simulink model "simulinkModelForOpenLoop"  (R2020b)
settings: Solver=VariableStepAuto  StartTime=0.0  StopTime=10.0  RelTol=1e-3
settings Model: Creator=saumya  LastModifiedBy=saumya

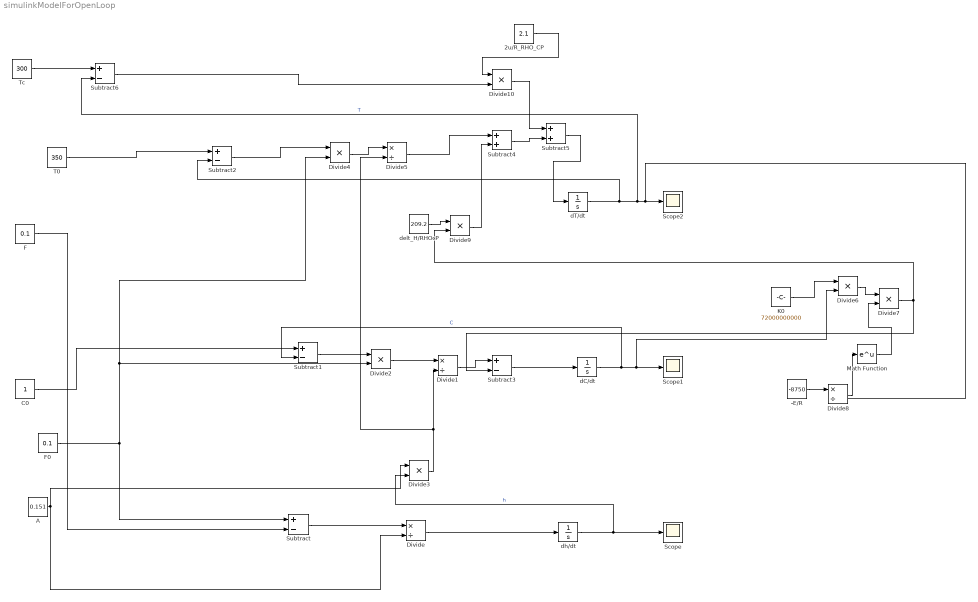
== system simulinkModelForOpenLoop ==
  -E/R : Constant  Value=-8750
  2u/R_RHO_CP : Constant  Value=2.1
  A : Constant  Value=0.151
  C0 : Constant
  Divide{,1,5,8} (4 alike) : Product  Inputs=*/
  Divide{2..4,6..7,9..10} (7 alike) : Product  Inputs=**
  F : Constant  Value=0.1
  F0 : Constant  Value=0.1
  K0 : Constant  Value=72000000000
  Math Function : Math  SaturateOnIntegerOverflow=on
  Scope : Scope
  Scope1 : Scope
  Scope2 : Scope
  Subtract{,1..3,6} (5 alike) : Sum  Inputs=+-
  Subtract4 : Sum
  Subtract5 : Sum
  T0 : Constant  Value=350
  Tc : Constant  Value=300
  dC/dt : Integrator
  dT/dt : Integrator
  delt_H/RHOcP : Constant  Value=209.2
  dh/dt : Integrator  InitialCondition=0.8
  wires:
  -E/R/1 -> Divide8/1
  Divide5/1 -> Subtract4/1
  Subtract/1 -> Divide/1
  Math Function/1 -> Divide7/2
  Subtract5/1 -> dT/dt/1
  dT/dt/1 -> Subtract2/2, Subtract6/2, Scope2/1, Divide8/2  "T"
  Subtract4/1 -> Subtract5/2
  2u/R_RHO_CP/1 -> Divide10/1
  Subtract1/1 -> Divide2/1
  delt_H/RHOcP/1 -> Divide9/1
  dh/dt/1 -> Scope/1, Divide3/2  "h"
  Divide9/1 -> Subtract4/2
  F/1 -> Subtract/2
  Subtract6/1 -> Divide10/2
  A/1 -> Divide/2, Divide3/1
  K0/1 -> Divide6/1
  dC/dt/1 -> Subtract1/2, Scope1/1, Divide6/2  "C"
  Divide3/1 -> Divide5/2, Divide1/2
  F0/1 -> Divide4/2, Divide2/2, Subtract/1
  Divide10/1 -> Subtract5/1
  Subtract3/1 -> dC/dt/1
  Divide/1 -> dh/dt/1
  Divide4/1 -> Divide5/1
  Divide6/1 -> Divide7/1
  Divide2/1 -> Divide1/1
  Subtract2/1 -> Divide4/1
  C0/1 -> Subtract1/1
  T0/1 -> Subtract2/1
  Divide7/1 -> Subtract3/2, Divide9/2
  Divide8/1 -> Math Function/1
  Divide1/1 -> Subtract3/1
  Tc/1 -> Subtract6/1
